simulink model "control_exam_"  (R2023a)
settings: Solver=VariableStepAuto  StartTime=0.0  StopTime=10.0  RelTol=1e-3
settings Model: Creator=hwayoungkim  LastModifiedBy=hwayoungkim

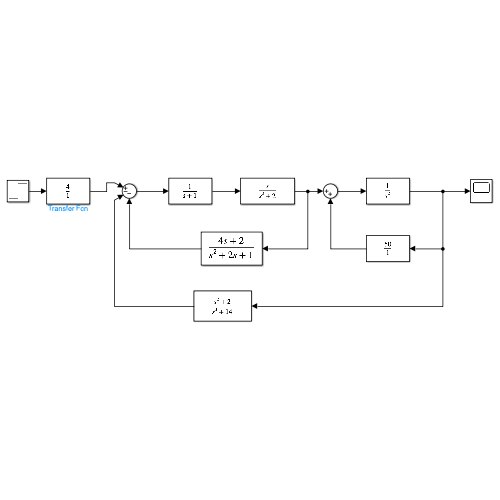
[thumbnail: Simulink's stored preview of the top-level diagram]
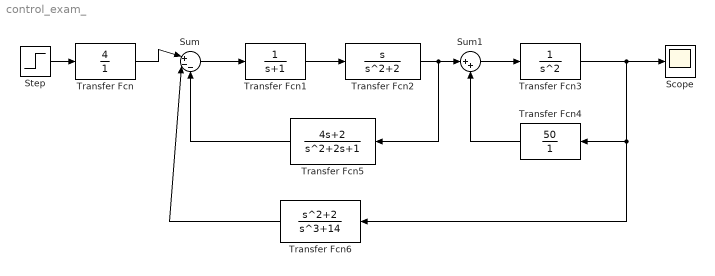
== system control_exam_ ==
  Scope : Scope
  Step : Step  SampleTime=0
  Sum : Sum  Inputs=|+--
  Sum1 : Sum  Inputs=|++
  Transfer Fcn : TransferFcn  Numerator=[4]  Denominator=[1]
  Transfer Fcn1 : TransferFcn  Denominator=[1 1]
  Transfer Fcn2 : TransferFcn  Numerator=[1 0]  Denominator=[1 0 2]
  Transfer Fcn3 : TransferFcn  Denominator=[1 0 0]
  Transfer Fcn4 : TransferFcn  Numerator=[50]  Denominator=[1]
  Transfer Fcn5 : TransferFcn  Numerator=[4 2]
  Transfer Fcn6 : TransferFcn  Numerator=[1 0 2]  Denominator=[1 0 0 14]
  wires:
  Transfer Fcn/1 -> Sum/1
  Sum/1 -> Transfer Fcn1/1
  Step/1 -> Transfer Fcn/1
  Transfer Fcn3/1 -> Transfer Fcn4/1, Transfer Fcn6/1, Scope/1
  Transfer Fcn1/1 -> Transfer Fcn2/1
  Transfer Fcn2/1 -> Transfer Fcn5/1, Sum1/1
  Sum1/1 -> Transfer Fcn3/1
  Transfer Fcn4/1 -> Sum1/2
  Transfer Fcn5/1 -> Sum/3
  Transfer Fcn6/1 -> Sum/2
